simulink model "tc387_xcp_demo"  (R2026a)
settings: Solver=FixedStepDiscrete  StopTime=10  FixedStep=0.001
undefined symbols (not defined in the file): FOC_20kHz, g_adc_raw_curr_u, g_adc_raw_curr_v, g_adc_raw_curr_w, g_adc_raw_res_cos, g_adc_raw_res_sin, g_duty_u, g_duty_v, g_duty_w, g_foc_exec_time_us, g_foc_isr_counter, g_meas_curr_u, g_meas_curr_v, g_meas_curr_w, g_meas_speed, g_meas_theta_mech, g_pwm_cm1_u, g_pwm_cm1_v, g_pwm_cm1_w
libraries: xcpprotocollib x2
settings Model: Creator=probst  LastModifiedBy=probst

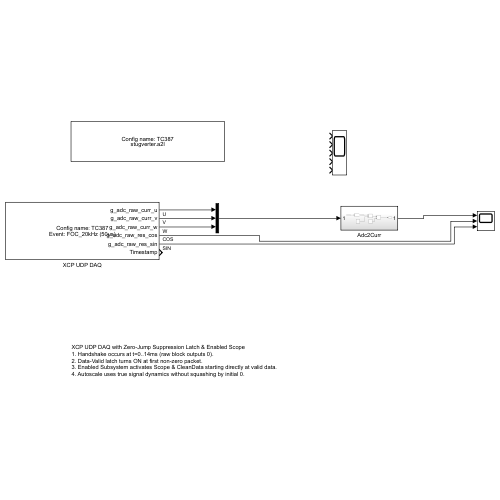
[thumbnail: Simulink's stored preview of the top-level diagram]
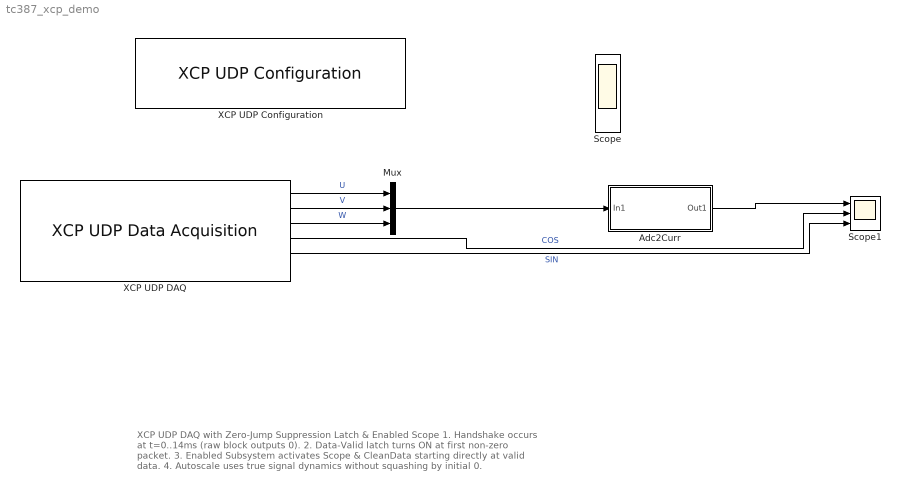
== system tc387_xcp_demo ==
  note: XCP UDP DAQ with Zero-Jump Suppression Latch & Enabled Scope
      | 1. Handshake occurs at t=0..14ms (raw block outputs 0).
      | 2. Data-Valid latch turns ON at first non-zero packet.
      | 3. Enabled Subsystem activates Scope & CleanData starting directly at valid data.
      | 4. Autoscale uses true signal dynamics without squashing by initial 0.
  Adc2Curr : Subsystem
  Mux : Mux  Inputs=3
  Scope : Scope  NumInputPorts=5
      settings: ActiveDisplayYMinimum=2226.887910798122  ActiveDisplayYMaximum=2248.85582942097
  Scope1 : Scope  NumInputPorts=3
      settings: ActiveDisplayYMinimum=1669  ActiveDisplayYMaximum=2449
  XCP UDP Configuration : xcpprotocollib/UDP/XCP UDP Configuration  Priority=-100  SlaveName=TC387  SlaveID=1  A2LFile=c:\Users\probst\Desktop\stugverter\firmware\stugverter.a2l  EnableSecurity=off  ConnectMode=off  EnableStatus=off  SampleTime=0.001  HeaderErrDet=on  CTRScheme=One counter for all CTOs and DTOs  LocalAddress=auto  LocalPort=auto  DAQTimeout=2
      settings: LibrarySourceBlock=vntxcplib/UDP/XCP UDP Configuration
  XCP UDP DAQ : xcpprotocollib/UDP/XCP UDP Data Acquisition  SlaveName=TC387  A2LFile=c:\Users\probst\Desktop\stugverter\firmware\stugverter.a2l  EventName=FOC_20kHz (50us)  AllMeasurements=g_adc_raw_curr_u;g_adc_raw_curr_v;g_adc_raw_curr_w;g_adc_raw_res_cos;g_adc_raw_res_sin;g_duty_u;g_duty_v;g_duty_w;g_foc_exec_time_us;g_foc_isr_counter;g_meas_curr_u;g_meas_curr_v;g_meas_curr_w;g_meas_speed;g_meas_theta_mech;g_pwm_cm1_u;g_pwm_cm1_v;g_pwm_cm1_w  SelectedMeasurements=g_adc_raw_curr_u;g_adc_raw_curr_v;g_adc_raw_curr_w;g_adc_raw_res_cos;g_adc_raw_res_sin  DAQPriority=0  SampleTime=0.001  EnableTimestamp=on  InputOrOutputDatatype=Raw values as double (no Compu method conversion)
      settings: LibrarySourceBlock=vntxcplib/UDP/XCP UDP Data Acquisition
  wires:
  XCP UDP DAQ/1 -> Mux/1  "U"
  Adc2Curr/1(Out1) -> Scope1/1
  Mux/1 -> Adc2Curr/1(In1)
  XCP UDP DAQ/2 -> Mux/2  "V"
  XCP UDP DAQ/3 -> Mux/3  "W"
  XCP UDP DAQ/4 -> Scope1/2  "COS"
  XCP UDP DAQ/5 -> Scope1/3  "SIN"

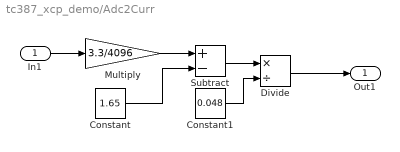
== system tc387_xcp_demo/Adc2Curr ==
  In1 : Inport
  Constant : Constant  Value=1.65
  Constant1 : Constant  Value=0.048
  Divide : Product  Inputs=*/
  Multiply : Gain  Gain=3.3/4096
  Subtract : Sum  Inputs=+-
  Out1 : Outport
  wires:
  In1/1 -> Multiply/1
  Multiply/1 -> Subtract/1
  Constant/1 -> Subtract/2
  Subtract/1 -> Divide/1
  Constant1/1 -> Divide/2
  Divide/1 -> Out1/1
